simulink model "Schema_inversione_cinematica_con_trasposta_Jacobiano"  (R2023a)
settings: Solver=VariableStepAuto  StartTime=0.0  StopTime=113  RelTol=1e-3
values from neighbouring files (symbols this model uses):
  a1 = 0.5    [Progetto_FoR.m]
  d0 = 1    [Progetto_FoR.m]
  KT = diag(kt)    [Progetto_FoR.m]
  q0 = [0 pi/2 0 pi/2]    [Progetto_FoR.m]
  Tc = 0.001    [Progetto_FoR.m]
undefined symbols (not defined in the file or in its folder): DiscIntNeverNeededParam
settings Model: Creator=panto  LastModifiedBy=panto

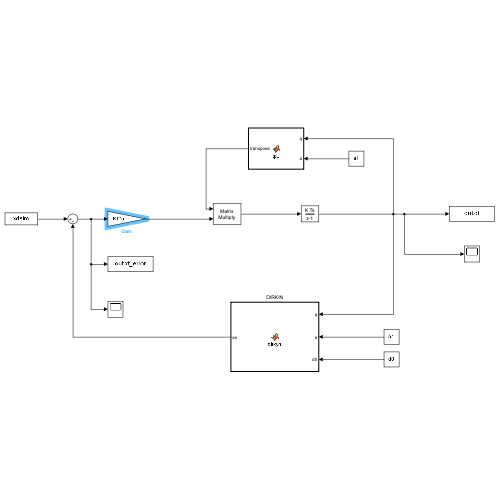
[thumbnail: Simulink's stored preview of the top-level diagram]
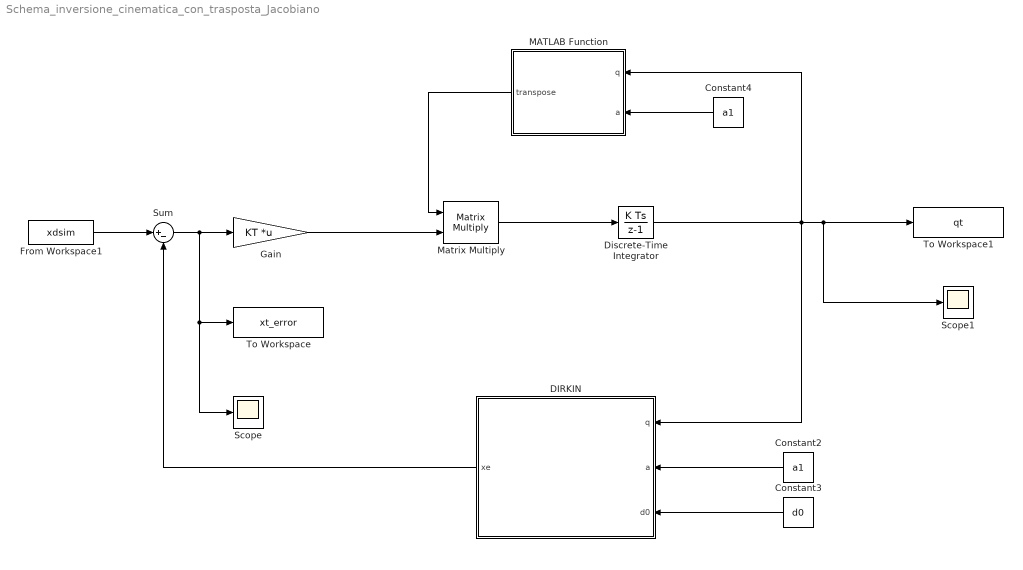
== system Schema_inversione_cinematica_con_trasposta_Jacobiano ==
  Constant2 : Constant  Value=a1
  Constant3 : Constant  Value=d0
  Constant4 : Constant  Value=a1
  DIRKIN : MATLAB Function  TreatAsAtomicUnit=on
  Discrete-Time Integrator : DiscreteIntegrator  InitialCondition=q0'  SampleTime=Tc  ICPrevOutput=DiscIntNeverNeededParam  ICPrevScaledInput=DiscIntNeverNeededParam
  From Workspace1 : FromWorkspace  VariableName=xdsim  SampleTime=Tc
  Gain : Gain  Gain=KT  Multiplication=Matrix(K*u)
  MATLAB Function : MATLAB Function  TreatAsAtomicUnit=on
  Matrix Multiply : Product  Multiplication=Matrix(*)
  Scope : Scope
  Scope1 : Scope
  Sum : Sum  Inputs=|+-
  To Workspace : ToWorkspace  VariableName=xt_error  SampleTime=Tc
      settings: Save2DSignal=2-D array (concatenate along first dimension)
  To Workspace1 : ToWorkspace  VariableName=qt  SampleTime=Tc
      settings: Save2DSignal=2-D array (concatenate along first dimension)
  wires:
  Discrete-Time Integrator/1 -> Scope1/1, To Workspace1/1, DIRKIN/1(q), MATLAB Function/1(q)
  Matrix Multiply/1 -> Discrete-Time Integrator/1
  Constant4/1 -> MATLAB Function/2(a)
  Constant3/1 -> DIRKIN/3(d0)
  MATLAB Function/1(transpose) -> Matrix Multiply/1
  DIRKIN/1(xe) -> Sum/2
  Constant2/1 -> DIRKIN/2(a)
  From Workspace1/1 -> Sum/1
  Sum/1 -> To Workspace/1, Scope/1, Gain/1
  Gain/1 -> Matrix Multiply/2

== matlab function Schema_inversione_cinematica_con_trasposta_Jacobiano/DIRKIN ==
  data: q input; xe output; a input; d0 input
function xe = dirkyn(q, a, d0)
  xe = zeros(4,1);
    xe = [a*cos(q(1)+q(2))+a*cos(q(1));
        a*sin(q(1)+q(2))+a*sin(q(1));
        d0-q(3);
        q(1)+q(2)-q(4)];
end

== matlab function Schema_inversione_cinematica_con_trasposta_Jacobiano/MATLAB Function ==
  data: q input; transpose output; a input
function transpose = tpJ(q,a)
   
    Ja = zeros(4,4);
    Ja = [-a*sin(q(1)+q(2))-a*sin(q(1)) -a*sin(q(1)+q(2)) 0 0;
        a*cos(q(1)+q(2))+a*cos(q(1)) a*cos(q(1)+q(2)) 0 0;
        0 0 -1 0;
        1 1 0 -1];

    transpose = Ja';

end
